simulink model "inverted_pendulum"  (R2024b)
settings: Solver=VariableStepAuto  StartTime=0.0  StopTime=1.5  RelTol=1e-3
settings Model: Creator=Austinchao  LastModifiedBy=Austinchao

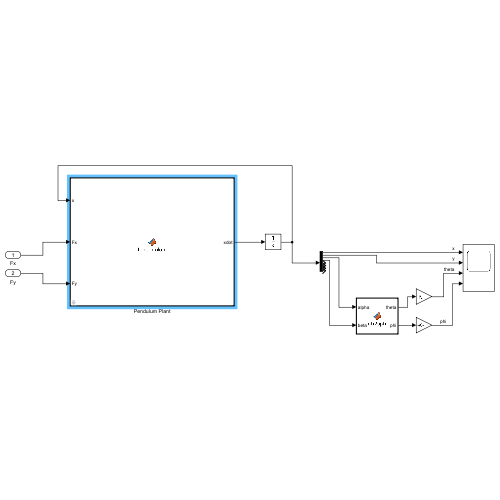
[thumbnail: Simulink's stored preview of the top-level diagram]
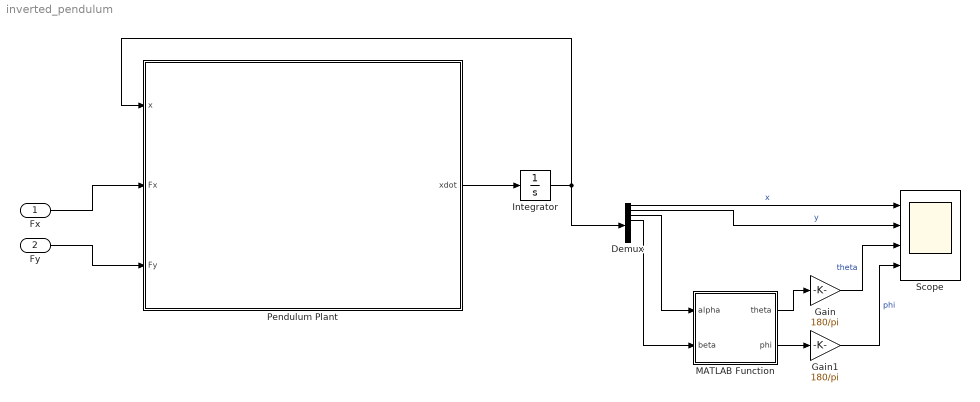
== system inverted_pendulum ==
  Fx : Inport
  Fy : Inport  Port=2
  Demux : Demux  Outputs=8
  Gain : Gain  Gain=180/pi
  Gain1 : Gain  Gain=180/pi
  Integrator : Integrator  InitialCondition=[0;0;deg2rad(5);deg2rad(-3);0;0;0;0]
  MATLAB Function : MATLAB Function  TreatAsAtomicUnit=on
  Pendulum Plant : MATLAB Function  TreatAsAtomicUnit=on  mask{m_pendulum=0.3, M_cart=5, l=0.6, g=9.81, Ipxx=0.05, Ipyy=0.05, Ipzz=0.05}
      mask prompts: m_pendulum "Pendulum mass (kg)"; M_cart "Chassis mass (kg)"; l "Rod Length (m)"; g "Gravity (m/s^2)"; Ipxx "Inertia Ixx"; Ipyy "Inertia Iyy"; Ipzz "Inertia Izz"
  Scope : Scope  NumInputPorts=4
  wires:
  Pendulum Plant/1(xdot) -> Integrator/1
  Integrator/1 -> Pendulum Plant/1(x), Demux/1
  Fx/1 -> Pendulum Plant/2(Fx)
  Fy/1 -> Pendulum Plant/3(Fy)
  Demux/1 -> Scope/1  "x"
  Demux/2 -> Scope/2  "y"
  Demux/3 -> MATLAB Function/1(alpha)
  Demux/4 -> MATLAB Function/2(beta)
  MATLAB Function/1(theta) -> Gain/1
  Gain/1 -> Scope/3  "theta"
  MATLAB Function/2(phi) -> Gain1/1
  Gain1/1 -> Scope/4  "phi"

== matlab function inverted_pendulum/MATLAB Function ==
  data: alpha input; theta output; beta input; phi output
function [theta, phi] = ab2sph(alpha, beta)
% alpha, beta : tilt angles in rad (projection angles wrt xz and yz planes)
% theta       : tilt magnitude (rad), 0 = upright, ~pi/2 = horizontal
% phi         : azimuth angle (rad), orientation in XY plane

% slope variables
ta = tan(alpha);
tb = tan(beta);

% azimuth angle (方向)
phi = atan2(tb, ta);

% tilt magnitude (傾斜大小)
theta = atan(sqrt(ta.^2 + tb.^2));

end

== matlab function inverted_pendulum/Pendulum Plant ==
  data: x input double size=[8 1]; xdot output double size=[8 1]; Fx input; Fy input; m_pendulum parameter; M_cart parameter; l parameter; g parameter; Ipxx parameter; Ipyy parameter; Ipzz parameter
function xdot = f_pendulum(x, Fx, Fy, m_pendulum, M_cart, l, g, Ipxx, Ipyy, Ipzz)
% x = [x; y; alpha; beta; dx; dy; dalpha; dbeta]

% Mask 參數 (會自動由 Mask GUI 傳入，不用 Inport)
% m_pendulum, M_cart, l, g, Ipxx, Ipyy, Ipzz

X   = x(1);   Y   = x(2);
a   = x(3);   b   = x(4);
dX  = x(5);   dY  = x(6);
da  = x(7);   db  = x(8);

% trig
cA = cos(a); sA = sin(a);
cB = cos(b); sB = sin(b);

% ----- Mass matrix M(q) -----
M11 = m_pendulum+M_cart;          M12 = m_pendulum*l*cA*cB;    M13 = 0;           M14 = -m_pendulum*l*sA*sB;
M21 = M12;                        M22 = m_pendulum*l^2*cB^2 + Ipyy*cB^2 + Ipzz*sB^2; M23 = 0; M24 = 0;
M31 = 0;                          M32 = 0;                     M33 = m_pendulum+M_cart; M34 = m_pendulum*l*cB;
M41 = -m_pendulum*l*sA*sB;        M42 = 0;                     M43 = m_pendulum*l*cB; M44 = m_pendulum*l^2 + Ipxx;

Mmat = [M11 M12 M13 M14;
        M21 M22 M23 M24;
        M31 M32 M33 M34;
        M41 M42 M43 M44];

% ----- h(q,dq) -----
h1 = (-m_pendulum*l*da*sA*cB - m_pendulum*db*cA*sB)*da + (-m_pendulum*db*sA*cB - m_pendulum*da*cA*sB)*db;
h2 = (-m_pendulum*l^2*db*sB*cB - Ipyy*db*sB*cB + Ipzz*db*sB*cB)*da ...
   + (-m_pendulum*l^2*da*sB*cB - Ipyy*da*sB*cB + Ipzz*da*sB*cB)*db ...
   - m_pendulum*g*l*sA*cB;
h3 = - m_pendulum*l*db^2*sB;
h4 = (m_pendulum*l^2*da*sB*cB + Ipyy*da*sB*cB - Ipzz*da*sB*cB)*da - m_pendulum*g*l*cA*sB;

h = [h1; h2; h3; h4];

% generalized forces
tau = [Fx; 0; Fy; 0];

% solve qdd
qdd = Mmat \ (tau - h);

% pack xdot = [dx; dy; dalpha; dbeta; ddx; ddy; ddalpha; ddbeta]
xdot = [dX; dY; da; db; qdd(1); qdd(3); qdd(2); qdd(4)];
end
